simulink model "robot"  (R2018a)
settings: Solver=VariableStepAuto  StartTime=0.0  StopTime=10  RelTol=1e-3
undefined symbols (not defined in the file or in its folder): X, Y, Z
libraries: sm_lib x40, nesl_utility x10, simulink x4
(part 2 of 2)

== matlab function robot/MATLAB Function ==
  data: x input; q1 output; y input; z input; q2 output; q3 output
function [q1,q2,q3] = fcn(x,y,z)
L1=0.5;
L2=0.6;
L3=0.35;

q1=atan2(y,x);
q2 = 2*atan((2*L2*(z - L1) - (L2^2*((- L2^2 + 2*L2*L3 - L3^2 + (x/cos((atan2(y,x))))^2 + (z - L1)^2)*(L2^2 + 2*L2*L3 + L3^2 - (x/cos((atan2(y,x))))^2 - (z - L1)^2))^(1/2))/(- L2^2 + 2*L2*L3 - L3^2 + (x/cos((atan2(y,x))))^2 + (z - L1)^2) - (L3^2*((- L2^2 + 2*L2*L3 - L3^2 + (x/cos((atan2(y,x))))^2 + (z - L1)^2)*(L2^2 + 2*L2*L3 + L3^2 - (x/cos((atan2(y,x))))^2 - (z - L1)^2))^(1/2))/(- L2^2 + 2*L2*L3 - L3^2 + (x/cos((atan2(y,x))))^2 + (z - L1)^2) + ((x/cos((atan2(y,x))))^2*((- L2^2 + 2*L2*L3 - L3^2 + (x/cos((atan2(y,x))))^2 + (z - L1)^2)*(L2^2 + 2*L2*L3 + L3^2 - (x/cos((atan2(y,x))))^2 - (z - L1)^2))^(1/2))/(- L2^2 + 2*L2*L3 - L3^2 + (x/cos((atan2(y,x))))^2 + (z - L1)^2) + ((z - L1)^2*((- L2^2 + 2*L2*L3 - L3^2 + (x/cos((atan2(y,x))))^2 + (z - L1)^2)*(L2^2 + 2*L2*L3 + L3^2 - (x/cos((atan2(y,x))))^2 - (z - L1)^2))^(1/2))/(- L2^2 + 2*L2*L3 - L3^2 + (x/cos((atan2(y,x))))^2 + (z - L1)^2) + (2*L2*L3*((- L2^2 + 2*L2*L3 - L3^2 + (x/cos((atan2(y,x))))^2 + (z - L1)^2)*(L2^2 + 2*L2*L3 + L3^2 - (x/cos((atan2(y,x))))^2 - (z - L1)^2))^(1/2))/(- L2^2 + 2*L2*L3 - L3^2 + (x/cos((atan2(y,x))))^2 + (z - L1)^2))/(L2^2 + 2*L2*(x/cos((atan2(y,x)))) - L3^2 + (x/cos((atan2(y,x))))^2 + (z - L1)^2));
q3 = -2*atan(((- L2^2 + 2*L2*L3 - L3^2 + (x/cos((atan2(y,x))))^2 + (z - L1)^2)*(L2^2 + 2*L2*L3 + L3^2 - (x/cos((atan2(y,x))))^2 - (z - L1)^2))^(1/2)/(- L2^2 + 2*L2*L3 - L3^2 + (x/cos((atan2(y,x))))^2 + (z - L1)^2));
end
